simulink model "SpeedgoatCANOpen07"  (R2018b)
settings: Solver=FixedStepDiscrete  StartTime=0.0  StopTime=inf  FixedStep=0.0001  RelTol=1e-3  EnableMultiTasking=on
libraries: slrtlib x9, speedgoatlib_IO691 x5
(part 1 of 2)
settings Model: DataDictionary=Trike_dictionary.sldd  SimulationMode=external  Creator=Venqo  LastModifiedBy=Venqo
settings SolverCC: ConcurrentTasks=on  AutoInsertRateTranBlk=on
settings DataIOCC: SaveFormat=StructureWithTime
settings OptimizationCC: BlockReduction=off  OptimizeBlockIOStorage=off  BufferReuse=off  GlobalBufferReuse=off  ExpressionFolding=off  LocalBlockOutputs=off  RollThreshold=10  OptimizeDataStoreBuffers=off  BusAssignmentInplaceUpdate=off
settings HardwareCC: ProdBitPerPointer=32  ProdBitPerSizeT=32  ProdBitPerPtrDiffT=32  ProdLargestAtomicFloat=None  ProdWordSize=32  ProdLongLongMode=on  ProdHWDeviceType=Generic->32-bit x86 compatible
settings SFSimCC: SimAnalyzeCustomCode=on
settings SFSimCC: SimCustomHeaderCode=|
  | #include "CANOpenSlave.h"
  | #include "CANOpenSlaveAPT.h"
settings SFSimCC: SimCustomInitializer=|
  | CANOpenSlave_ResetCommunication();
  | CANOpenSlave_ResetCommunication_APT();
settings SFSimCC: SimUserSources=|
  | CANOpenSlave.c
  | CANOpenSlaveAPT.c
settings RTWCC: SystemTargetFile=slrt.tlc  TemplateMakefile=slrt_default_tmf  Description=Simulink Real-Time  CodeExecutionProfiling=on  RTWCompilerOptimization=on
settings RTWCC: CustomHeaderCode=|
  | #include "CANOpenSlave.h"
  | #include "CANOpenSlaveAPT.h"
settings RTWCC: CustomSource=|
  | CANOpenSlave.c
  | CANOpenSlaveAPT.c
settings RTWCC: CustomInitializer=|
  | CANOpenSlave_ResetCommunication();
  | CANOpenSlave_ResetCommunication_APT();
settings SimulinkRealTimeCC: InferredTypesCompatibility=on  SupportVariableSizeSignals=on  PreserveStateflowLocalDataDimensions=off  RL32LogTETModifier=off  xPCConcurrentTasks=on

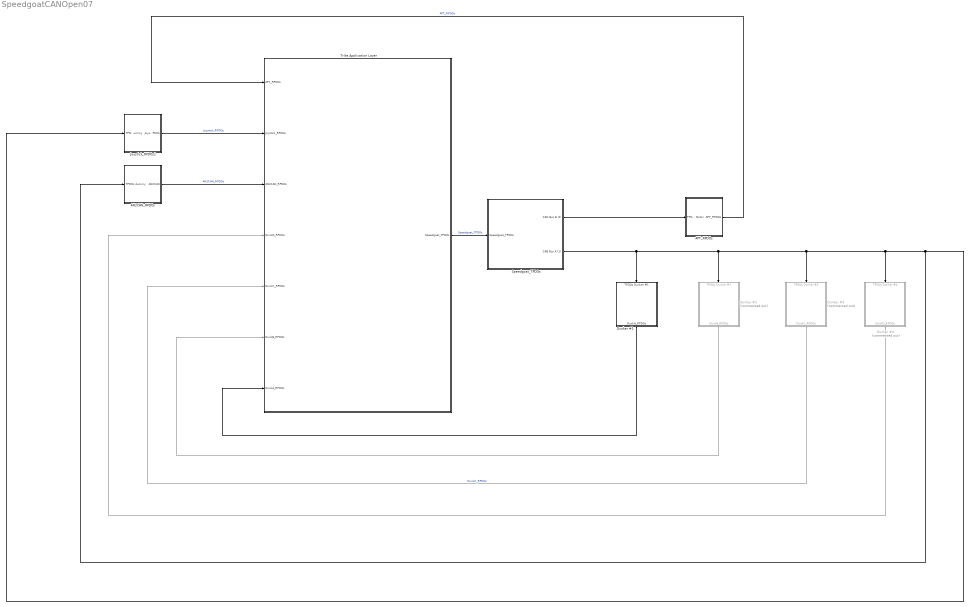
== system SpeedgoatCANOpen07 ==
  AN2CAN_RPDOs : Subsystem
      mask Display: image('C:\Users\Venqo\Desktop\SpeedGoat\Applications\Trike_01_2CANbuses\Img\mcan_box_4xi.png');
  APT_RPDOs : Subsystem
      mask Display: image('C:\Users\Venqo\Desktop\SpeedGoat\Applications\Trike_05\Img\aptqsmotor.png');
  Dunker #1 : Subsystem
      mask Display: image('C:\Users\Venqo\Desktop\SpeedGoat\Applications\Trike_01_2CANbuses\Img\dunk.png');
  Dunker #2 : Subsystem  Commented=on
      mask Display: image('C:\Users\Venqo\Desktop\SpeedGoat\Applications\Trike_01_2CANbuses\Img\dunk.png');
  Dunker #3 : Subsystem  Commented=on
      mask Display: image('C:\Users\Venqo\Desktop\SpeedGoat\Applications\Trike_01_2CANbuses\Img\dunk.png');
  Dunker #4 : Subsystem  Commented=on
      mask Display: image('C:\Users\Venqo\Desktop\SpeedGoat\Applications\Trike_01_2CANbuses\Img\dunk.png');
  Joystick_RPDOs1 : Subsystem
      mask Display: image('C:\Users\Venqo\Desktop\SpeedGoat\Applications\Trike_05\Img\joystick.png');
  Speedgoat_TPDOs : Subsystem
      mask Display: image('C:\Users\Venqo\Desktop\SpeedGoat\Applications\Trike_05\Img\speedgoat.png');
  Trike Application Layer : Subsystem
      mask Display: image('C:\Users\Venqo\Desktop\SpeedGoat\Applications\Trike_05\Img\trike.png');
  wires:
  Joystick_RPDOs1/1(Joystick_RPDOs) -> Trike Application Layer/2(Joystick_RPDOs)  "Joystick_RPDOs"
  Trike Application Layer/1(Speedgoat_TPDOs) -> Speedgoat_TPDOs/1(Speedgoat_TPDOs)  "Speedgoat_TPDOs"
  AN2CAN_RPDOs/1(AN2CAN) -> Trike Application Layer/3(AN2CAN_RPDOs)  "AN2CAN_RPDOs"
  Dunker #3/1(DunkC_RPDOs) -> Trike Application Layer/5(DunkC_RPDOs)  "DunkC_RPDOs"
  Dunker #1/1(DunkA_RPDOs) -> Trike Application Layer/7(DunkA_RPDOs)
  Dunker #2/1(DunkB_RPDOs) -> Trike Application Layer/6(DunkB_RPDOs)
  Dunker #4/1(DunkD_RPDOs) -> Trike Application Layer/4(DunkD_RPDOs)
  Speedgoat_TPDOs/1("CAN Bus B (2) ") -> APT_RPDOs/1("TPDOs APT - QS Motor ")
  APT_RPDOs/1(APT_RPDOs) -> Trike Application Layer/1(APT_RPDOs)  "APT_RPDOs"
  Speedgoat_TPDOs/2(CAB Bus A (1)) -> Dunker #1/1(TPDOs Dunker #1), Dunker #2/1(TPDOs Dunker #1), Dunker #3/1(TPDOs Dunker #3), Dunker #4/1(TPDOs Dunker #4), AN2CAN_RPDOs/1(TPDOs dummy), Joystick_RPDOs1/1(TPDOs dummy)

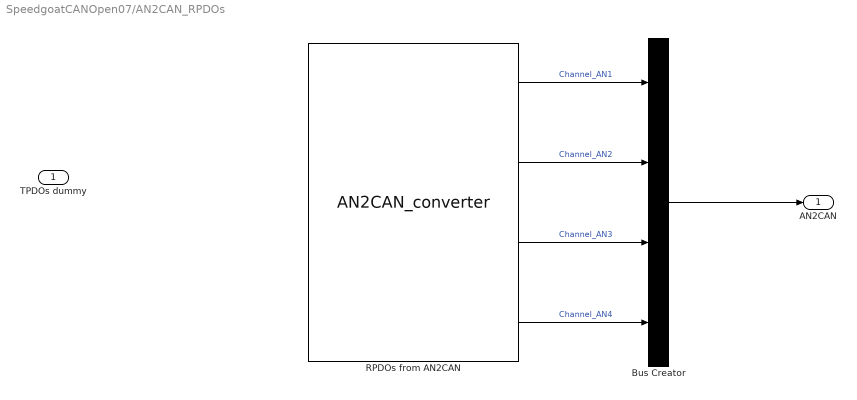
== system SpeedgoatCANOpen07/AN2CAN_RPDOs ==
  TPDOs dummy : Inport
  Bus Creator : BusCreator  Inputs=4  OutDataTypeStr=Bus: AN2CAN_conv
  "RPDOs from AN2CAN " : S-Function  InitFcn=try, set_param(gcb,'FunctionName','AN2CAN_converter'), end  FunctionName=AN2CAN_converter  SFunctionModules=AN2CAN_converter_wrapper  SFunctionDeploymentMode=off  EnableBusSupport=off  mask(S-Function Builder){}
      mask help: Simulink:masks:SFunctionBuilder_MD
      mask init:
      | val = [[.9  0.75 0.75 1 1 .9 .9 1]',[1 1 0.75 0.75 .9 .9 1 .9]'];try , sys = get_param(gcb,'SfunBuilderFcnName');if isempty(sys), sys = get_param(gcb,'FunctionName'); end,catch, sys = get_param(gcb,'FunctionName'); end
      settings: CopyFcn=set_param(gcbh,'LinkStatus','none')  PreSaveFcn=try, set_param(gcb,'FunctionName','AN2CAN_converter'), end  OpenFcn=sfunctionwizard(gcbh)
      mask Display: plot(val(:,1),val(:,2)),disp(sys), port_label('output',1,'Channel_AN1'), port_label('output',2,'Channel_AN2'), port_label('output',3,'Channel_AN3'), port_label('output',4,'Channel_AN4')
  AN2CAN : Outport  OutDataTypeStr=Bus: AN2CAN_conv
  wires:
  Bus Creator/1 -> AN2CAN/1
  "RPDOs from AN2CAN "/3 -> Bus Creator/3  "Channel_AN3"
  "RPDOs from AN2CAN "/4 -> Bus Creator/4  "Channel_AN4"
  "RPDOs from AN2CAN "/2 -> Bus Creator/2  "Channel_AN2"
  "RPDOs from AN2CAN "/1 -> Bus Creator/1  "Channel_AN1"

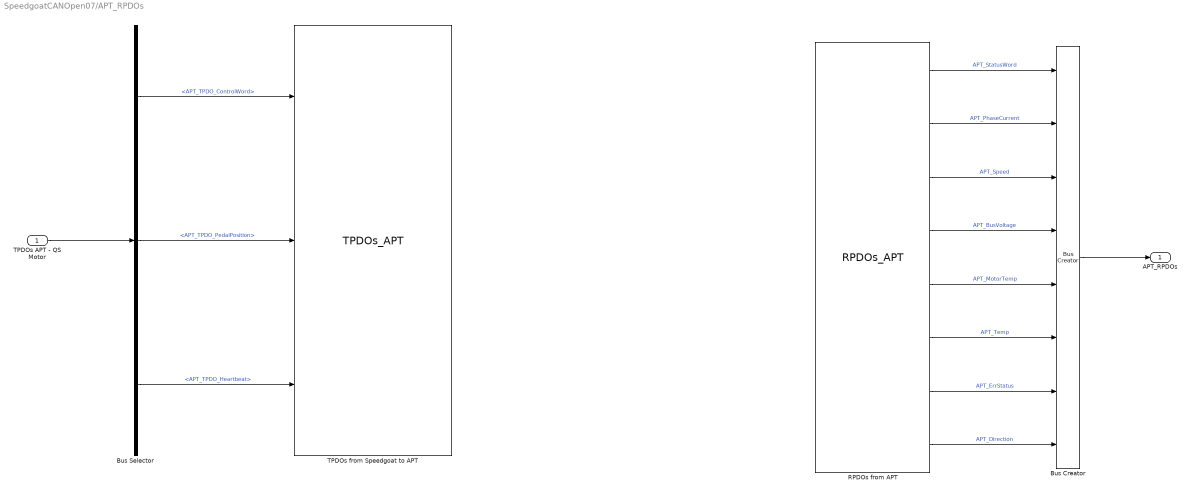
== system SpeedgoatCANOpen07/APT_RPDOs ==
  "TPDOs APT - QS Motor " : Inport
  Bus Creator : BusCreator  Inputs=8  OutDataTypeStr=Bus: APT_RPDOs
  Bus Selector : BusSelector  OutputSignals=APT_TPDO_ControlWord,APT_TPDO_PedalPosition,APT_TPDO_Heartbeat
  RPDOs from APT : S-Function  InitFcn=try, set_param(gcb,'FunctionName','RPDOs_APT'), end  FunctionName=RPDOs_APT  SFunctionModules=RPDOs_APT_wrapper  SFunctionDeploymentMode=off  EnableBusSupport=off  mask(S-Function Builder){}
      mask help: Simulink:masks:SFunctionBuilder_MD
      mask init: same as SpeedgoatCANOpen07/AN2CAN_RPDOs/RPDOs from AN2CAN 
      settings: CopyFcn=set_param(gcbh,'LinkStatus','none')  PreSaveFcn=try, set_param(gcb,'FunctionName','RPDOs_APT'), end  OpenFcn=sfunctionwizard(gcbh)
      mask Display: plot(val(:,1),val(:,2)),disp(sys), port_label('output',1,'StatusWord'), port_label('output',2,'PhaseCurrent'), port_label('output',3,'Speed'), port_label('output',4,'BusVoltage'), port_label('output',5,'MotorTemp'), port_label('output',6,'APTTemp'), port_label('output',7,'ErrStatus'), port_label('output',8,'Direction')
  TPDOs from Speedgoat to APT : S-Function  InitFcn=try, set_param(gcb,'FunctionName','TPDOs_APT'), end  FunctionName=TPDOs_APT  SFunctionModules=TPDOs_APT_wrapper  SFunctionDeploymentMode=off  EnableBusSupport=off  mask(S-Function Builder){}
      mask help: Simulink:masks:SFunctionBuilder_MD
      mask init: same as SpeedgoatCANOpen07/AN2CAN_RPDOs/RPDOs from AN2CAN 
      settings: CopyFcn=set_param(gcbh,'LinkStatus','none')  PreSaveFcn=try, set_param(gcb,'FunctionName','TPDOs_APT'), end  OpenFcn=sfunctionwizard(gcbh)
      mask Display: plot(val(:,1),val(:,2)),disp(sys), port_label('input',1,'APT_ControlWord'), port_label('input',2,'APT_PedalPosition'), port_label('input',3,'APT_HeartBeat')
  APT_RPDOs : Outport  OutDataTypeStr=Bus: APT_RPDOs
  wires:
  Bus Creator/1 -> APT_RPDOs/1
  RPDOs from APT/8 -> Bus Creator/8  "APT_Direction"
  RPDOs from APT/2 -> Bus Creator/2  "APT_PhaseCurrent"
  RPDOs from APT/6 -> Bus Creator/6  "APT_Temp"
  RPDOs from APT/3 -> Bus Creator/3  "APT_Speed"
  RPDOs from APT/1 -> Bus Creator/1  "APT_StatusWord"
  RPDOs from APT/5 -> Bus Creator/5  "APT_MotorTemp"
  RPDOs from APT/7 -> Bus Creator/7  "APT_ErrStatus"
  RPDOs from APT/4 -> Bus Creator/4  "APT_BusVoltage"
  "TPDOs APT - QS Motor "/1 -> Bus Selector/1
  Bus Selector/1 -> TPDOs from Speedgoat to APT/1  "<APT_TPDO_ControlWord>"
  Bus Selector/2 -> TPDOs from Speedgoat to APT/2  "<APT_TPDO_PedalPosition>"
  Bus Selector/3 -> TPDOs from Speedgoat to APT/3  "<APT_TPDO_Heartbeat>"

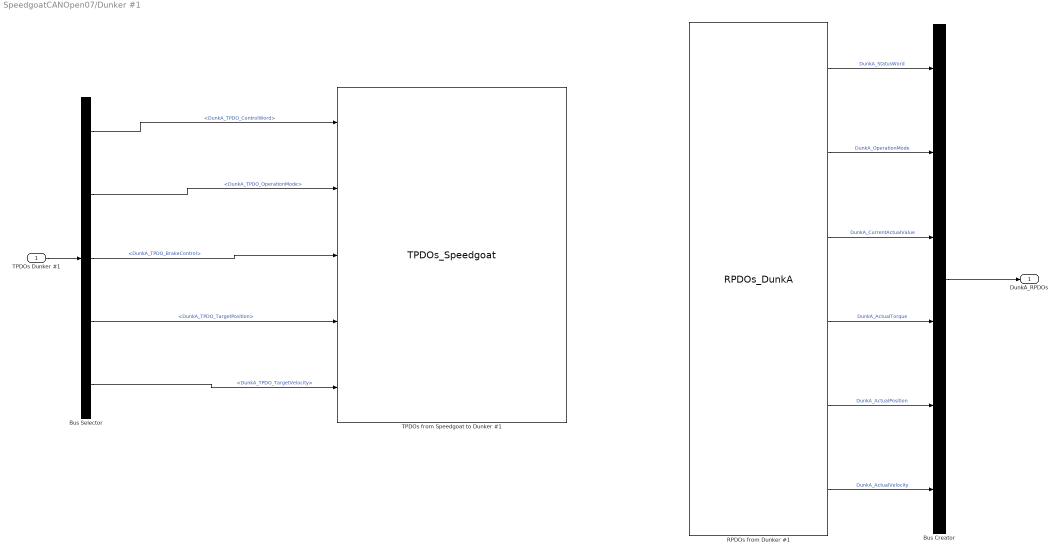
== system SpeedgoatCANOpen07/Dunker #1 ==
  TPDOs Dunker #1 : Inport
  Bus Creator : BusCreator  Inputs=6
  Bus Selector : BusSelector  OutputSignals=DunkA_TPDO_ControlWord,DunkA_TPDO_OperationMode,DunkA_TPDO_BrakeControl,DunkA_TPDO_TargetPosition,DunkA_TPDO_TargetVelocity
  RPDOs from Dunker #1 : S-Function  InitFcn=try, set_param(gcb,'FunctionName','RPDOs_DunkA'), end  FunctionName=RPDOs_DunkA  SFunctionModules=RPDOs_DunkA_wrapper  SFunctionDeploymentMode=off  EnableBusSupport=off  mask(S-Function Builder){}
      mask help: Simulink:masks:SFunctionBuilder_MD
      mask init: same as SpeedgoatCANOpen07/AN2CAN_RPDOs/RPDOs from AN2CAN 
      settings: CopyFcn=set_param(gcbh,'LinkStatus','none')  PreSaveFcn=try, set_param(gcb,'FunctionName','RPDOs_DunkA'), end  OpenFcn=sfunctionwizard(gcbh)
      mask Display: plot(val(:,1),val(:,2)),disp(sys), port_label('output',1,'StatusWord'), port_label('output',2,'OperationMode'), port_label('output',3,'CurrentActualValue'), port_label('output',4,'ActualTorque'), port_label('output',5,'ActualPosition'), port_label('output',6,'ActualVelocity')
  TPDOs from Speedgoat to Dunker #1 : S-Function  InitFcn=try, set_param(gcb,'FunctionName','TPDOs_Speedgoat'), end  FunctionName=TPDOs_Speedgoat  SFunctionModules=TPDOs_Speedgoat_wrapper  SFunctionDeploymentMode=off  EnableBusSupport=off  mask(S-Function Builder){}
      mask help: Simulink:masks:SFunctionBuilder_MD
      mask init: same as SpeedgoatCANOpen07/AN2CAN_RPDOs/RPDOs from AN2CAN 
      settings: CopyFcn=set_param(gcbh,'LinkStatus','none')  PreSaveFcn=try, set_param(gcb,'FunctionName','TPDOs_Speedgoat'), end  OpenFcn=sfunctionwizard(gcbh)
      mask Display: plot(val(:,1),val(:,2)),disp(sys), port_label('input',1,'DunkA_ControlWord'), port_label('input',2,'DunkA_OperationMode'), port_label('input',3,'DunkA_BrakeControl'), port_label('input',4,'DunkA_TargetPosition'), port_label('input',5,'DunkA_TargetVelocity')
  DunkA_RPDOs : Outport
  wires:
  Bus Selector/2 -> TPDOs from Speedgoat to Dunker #1/2  "<DunkA_TPDO_OperationMode>"
  Bus Selector/5 -> TPDOs from Speedgoat to Dunker #1/5  "<DunkA_TPDO_TargetVelocity>"
  TPDOs Dunker #1/1 -> Bus Selector/1
  Bus Selector/4 -> TPDOs from Speedgoat to Dunker #1/4  "<DunkA_TPDO_TargetPosition>"
  Bus Selector/1 -> TPDOs from Speedgoat to Dunker #1/1  "<DunkA_TPDO_ControlWord>"
  Bus Selector/3 -> TPDOs from Speedgoat to Dunker #1/3  "<DunkA_TPDO_BrakeControl>"
  RPDOs from Dunker #1/6 -> Bus Creator/6  "DunkA_ActualVelocity"
  Bus Creator/1 -> DunkA_RPDOs/1
  RPDOs from Dunker #1/1 -> Bus Creator/1  "DunkA_StatusWord"
  RPDOs from Dunker #1/4 -> Bus Creator/4  "DunkA_ActualTorque"
  RPDOs from Dunker #1/2 -> Bus Creator/2  "DunkA_OperationMode"
  RPDOs from Dunker #1/3 -> Bus Creator/3  "DunkA_CurrentActualValue"
  RPDOs from Dunker #1/5 -> Bus Creator/5  "DunkA_ActualPosition"

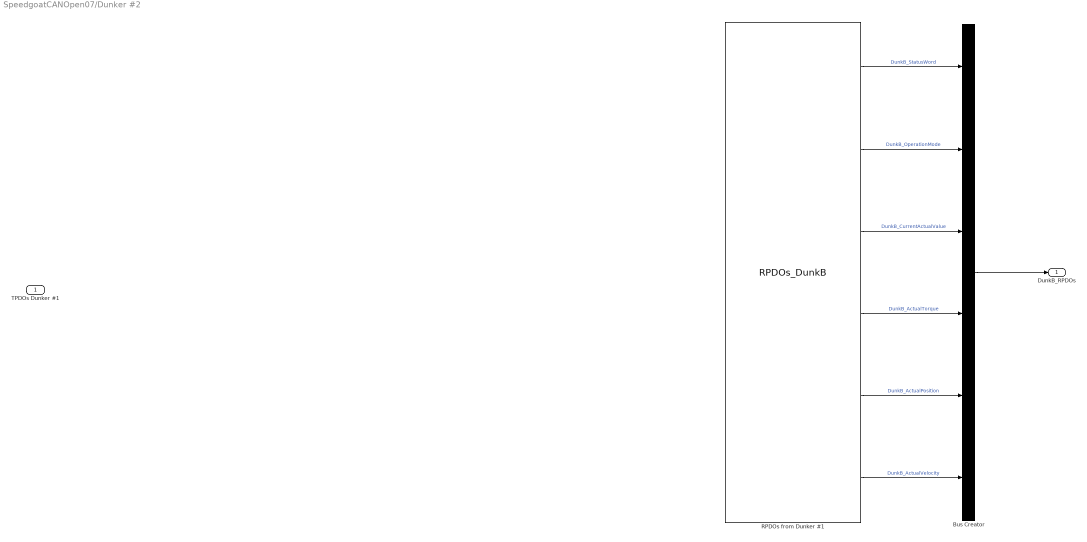
== system SpeedgoatCANOpen07/Dunker #2 ==
  TPDOs Dunker #1 : Inport
  Bus Creator : BusCreator  Inputs=6
  RPDOs from Dunker #1 : S-Function  InitFcn=try, set_param(gcb,'FunctionName','RPDOs_DunkB'), end  FunctionName=RPDOs_DunkB  SFunctionModules=RPDOs_DunkB_wrapper  SFunctionDeploymentMode=off  EnableBusSupport=off  mask(S-Function Builder){}
      mask help: Simulink:masks:SFunctionBuilder_MD
      mask init: same as SpeedgoatCANOpen07/AN2CAN_RPDOs/RPDOs from AN2CAN 
      settings: CopyFcn=set_param(gcbh,'LinkStatus','none')  PreSaveFcn=try, set_param(gcb,'FunctionName','RPDOs_DunkB'), end  OpenFcn=sfunctionwizard(gcbh)
      mask Display: plot(val(:,1),val(:,2)),disp(sys), port_label('output',1,'StatusWord'), port_label('output',2,'OperationMode'), port_label('output',3,'CurrentActualValue'), port_label('output',4,'ActualTorque'), port_label('output',5,'ActualPosition'), port_label('output',6,'ActualVelocity')
  DunkB_RPDOs : Outport
  wires:
  RPDOs from Dunker #1/1 -> Bus Creator/1  "DunkB_StatusWord"
  RPDOs from Dunker #1/3 -> Bus Creator/3  "DunkB_CurrentActualValue"
  RPDOs from Dunker #1/6 -> Bus Creator/6  "DunkB_ActualVelocity"
  RPDOs from Dunker #1/4 -> Bus Creator/4  "DunkB_ActualTorque"
  RPDOs from Dunker #1/5 -> Bus Creator/5  "DunkB_ActualPosition"
  Bus Creator/1 -> DunkB_RPDOs/1
  RPDOs from Dunker #1/2 -> Bus Creator/2  "DunkB_OperationMode"

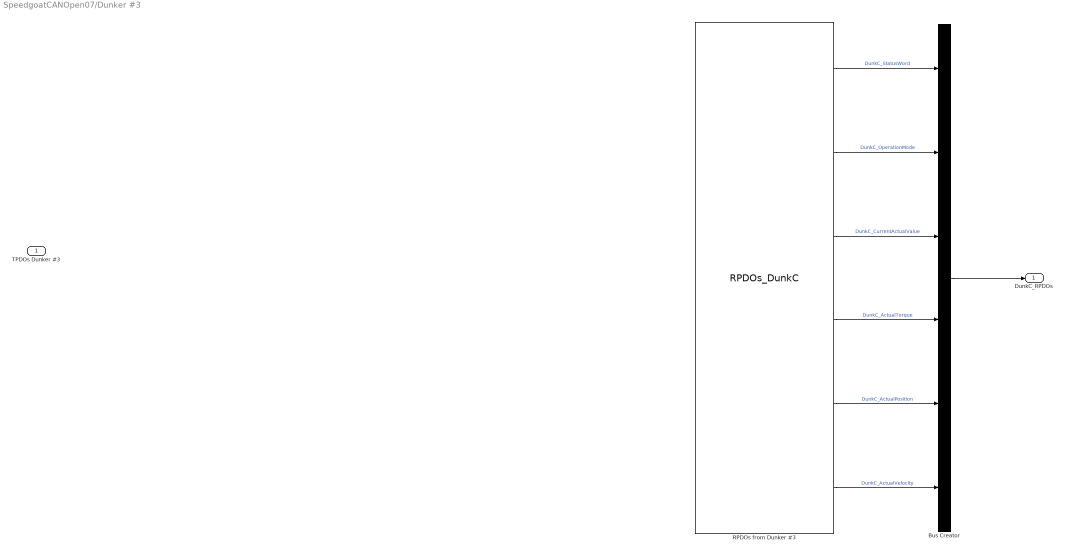
== system SpeedgoatCANOpen07/Dunker #3 ==
  TPDOs Dunker #3 : Inport
  Bus Creator : BusCreator  Inputs=6
  RPDOs from Dunker #3 : S-Function  InitFcn=try, set_param(gcb,'FunctionName','RPDOs_DunkC'), end  FunctionName=RPDOs_DunkC  SFunctionModules=RPDOs_DunkC_wrapper  SFunctionDeploymentMode=off  EnableBusSupport=off  mask(S-Function Builder){}
      mask help: Simulink:masks:SFunctionBuilder_MD
      mask init: same as SpeedgoatCANOpen07/AN2CAN_RPDOs/RPDOs from AN2CAN 
      settings: CopyFcn=set_param(gcbh,'LinkStatus','none')  PreSaveFcn=try, set_param(gcb,'FunctionName','RPDOs_DunkC'), end  OpenFcn=sfunctionwizard(gcbh)
      mask Display: plot(val(:,1),val(:,2)),disp(sys), port_label('output',1,'StatusWord'), port_label('output',2,'OperationMode'), port_label('output',3,'CurrentActualValue'), port_label('output',4,'ActualTorque'), port_label('output',5,'ActualPosition'), port_label('output',6,'ActualVelocity')
  DunkC_RPDOs : Outport
  wires:
  Bus Creator/1 -> DunkC_RPDOs/1
  RPDOs from Dunker #3/3 -> Bus Creator/3  "DunkC_CurrentActualValue"
  RPDOs from Dunker #3/5 -> Bus Creator/5  "DunkC_ActualPosition"
  RPDOs from Dunker #3/4 -> Bus Creator/4  "DunkC_ActualTorque"
  RPDOs from Dunker #3/1 -> Bus Creator/1  "DunkC_StatusWord"
  RPDOs from Dunker #3/2 -> Bus Creator/2  "DunkC_OperationMode"
  RPDOs from Dunker #3/6 -> Bus Creator/6  "DunkC_ActualVelocity"

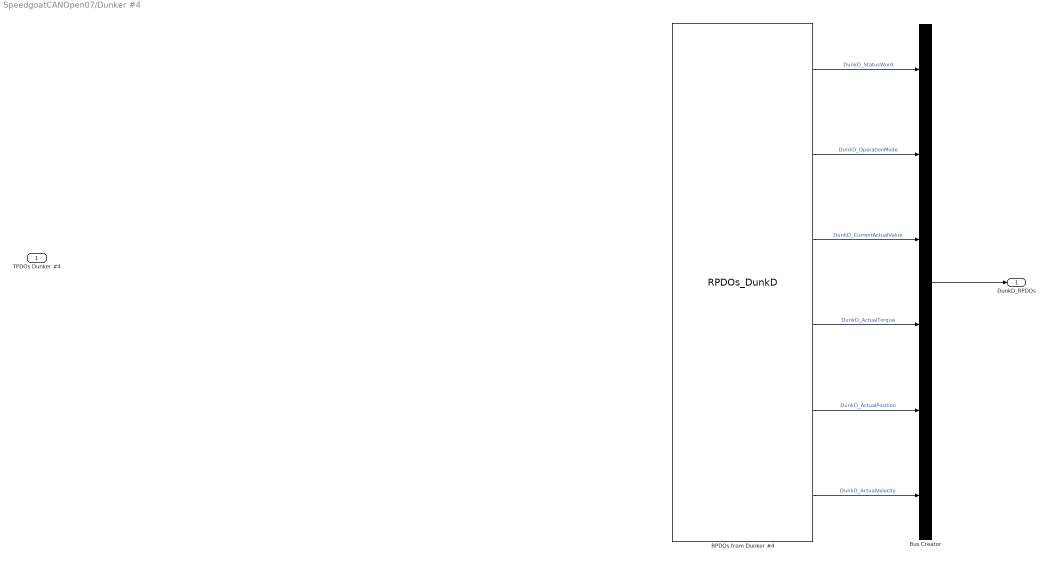
== system SpeedgoatCANOpen07/Dunker #4 ==
  TPDOs Dunker #4 : Inport
  Bus Creator : BusCreator  Inputs=6
  RPDOs from Dunker #4 : S-Function  InitFcn=try, set_param(gcb,'FunctionName','RPDOs_DunkD'), end  FunctionName=RPDOs_DunkD  SFunctionModules=RPDOs_DunkD_wrapper  SFunctionDeploymentMode=off  EnableBusSupport=off  mask(S-Function Builder){}
      mask help: Simulink:masks:SFunctionBuilder_MD
      mask init: same as SpeedgoatCANOpen07/AN2CAN_RPDOs/RPDOs from AN2CAN 
      settings: CopyFcn=set_param(gcbh,'LinkStatus','none')  PreSaveFcn=try, set_param(gcb,'FunctionName','RPDOs_DunkD'), end  OpenFcn=sfunctionwizard(gcbh)
      mask Display: plot(val(:,1),val(:,2)),disp(sys), port_label('output',1,'StatusWord'), port_label('output',2,'OperationMode'), port_label('output',3,'CurrentActualValue'), port_label('output',4,'ActualTorque'), port_label('output',5,'ActualPosition'), port_label('output',6,'ActualVelocity')
  DunkD_RPDOs : Outport
  wires:
  Bus Creator/1 -> DunkD_RPDOs/1
  RPDOs from Dunker #4/1 -> Bus Creator/1  "DunkD_StatusWord"
  RPDOs from Dunker #4/5 -> Bus Creator/5  "DunkD_ActualPosition"
  RPDOs from Dunker #4/4 -> Bus Creator/4  "DunkD_ActualTorque"
  RPDOs from Dunker #4/3 -> Bus Creator/3  "DunkD_CurrentActualValue"
  RPDOs from Dunker #4/6 -> Bus Creator/6  "DunkD_ActualVelocity"
  RPDOs from Dunker #4/2 -> Bus Creator/2  "DunkD_OperationMode"

== system SpeedgoatCANOpen07/Joystick_RPDOs1 ==
  TPDOs dummy : Inport
  Bus Creator : BusCreator  Inputs=3  OutDataTypeStr=Bus: Joystick_RPDOs
  RPDOs from Joystick : S-Function  InitFcn=try, set_param(gcb,'FunctionName','RPDOs_Joystick'), end  FunctionName=RPDOs_Joystick  SFunctionModules=RPDOs_Joystick_wrapper  SFunctionDeploymentMode=off  EnableBusSupport=off  mask(S-Function Builder){}
      mask help: Simulink:masks:SFunctionBuilder_MD
      mask init: same as SpeedgoatCANOpen07/AN2CAN_RPDOs/RPDOs from AN2CAN 
      settings: CopyFcn=set_param(gcbh,'LinkStatus','none')  PreSaveFcn=try, set_param(gcb,'FunctionName','RPDOs_Joystick'), end  OpenFcn=sfunctionwizard(gcbh)
      mask Display: plot(val(:,1),val(:,2)),disp(sys), port_label('output',1,'ButtonsStatus'), port_label('output',2,'LongCmd'), port_label('output',3,'LatCmd')
  Joystick_RPDOs : Outport  OutDataTypeStr=Bus: Joystick_RPDOs
  wires:
  RPDOs from Joystick/3 -> Bus Creator/3  "Joystick_LatCmd"
  RPDOs from Joystick/2 -> Bus Creator/2  "Joystick_LongCmd"
  RPDOs from Joystick/1 -> Bus Creator/1  "Joystick_ButtonsStatus"
  Bus Creator/1 -> Joystick_RPDOs/1

== system SpeedgoatCANOpen07/Speedgoat_TPDOs ==
  Speedgoat_TPDOs : Inport  OutDataTypeStr=Bus: Speedgoat_TPDOs
  CAN Bus Communication : Subsystem
  "CAN Bus B (2) " : Outport
  CAB Bus A (1) : Outport  Port=2
  wires:
  Speedgoat_TPDOs/1 -> CAB Bus A (1)/1, "CAN Bus B (2) "/1

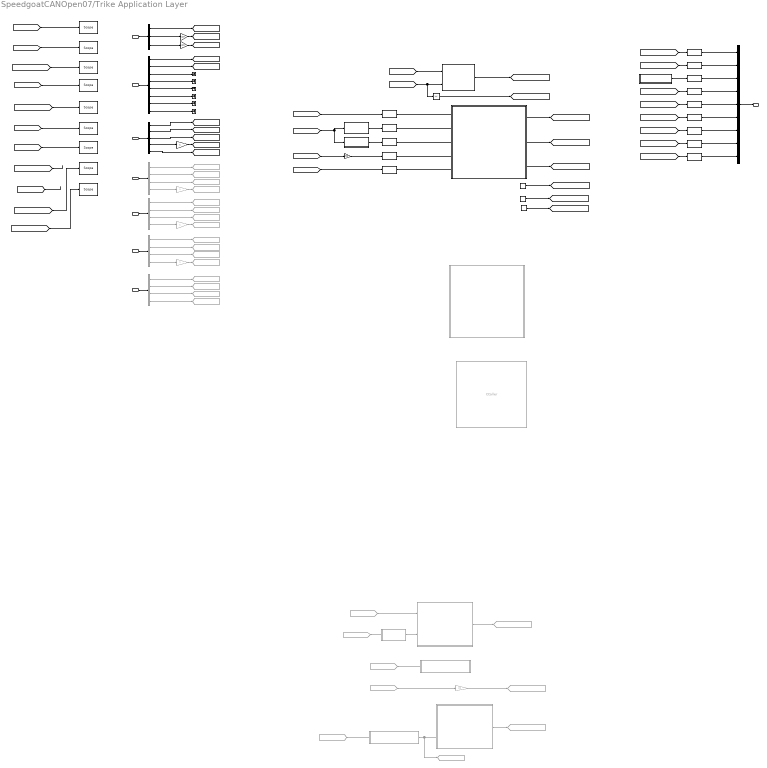
== system SpeedgoatCANOpen07/Trike Application Layer ==
  note: Speedgoat TPDOs / Control
  note: Speedgoat_Scopes
  note: RPDOs from Trike / Feedbacks
  APT_RPDOs : Inport  OutDataTypeStr=Bus: APT_RPDOs
  Joystick_RPDOs : Inport  Port=2  OutDataTypeStr=Bus: Joystick_RPDOs
  AN2CAN_RPDOs : Inport  Port=3  OutDataTypeStr=Bus: AN2CAN_conv
  DunkD_RPDOs : Inport  Port=4
  DunkC_RPDOs : Inport  Port=5
  DunkB_RPDOs : Inport  Port=6
  DunkA_RPDOs : Inport  Port=7
  APT BusVoltage : slrtlib/Displays and Logging/Scope   scopeno=3  scopetype=Target  autostart=on  viewmode=Graphical sliding  formatstr='%15.6f'  grid=on  ylimits=[0,130]  nosamples=50000  noprepostsamples=0  interleave=1  triggermode=FreeRun  triggersignal=1  trigsignalfromport=off  triggerlevel=0.0  triggerslope=Rising  triggerscope=1  triggersample=0  filename=data.dat  mode=Lazy  writesize=512  autorestart=off  dynamicfilemode=off  maxwritefilesize=512*1024^2
  Abs : Abs
  Bus Creator : BusCreator  Inputs=9  OutDataTypeStr=Bus: Speedgoat_TPDOs
  Bus Selector : BusSelector  OutputSignals=Joystick_ButtonsStatus,Joystick_LongCmd,Joystick_LatCmd
  Bus Selector1 : BusSelector  OutputSignals=APT_StatusWord,APT_PhaseCurrent,APT_Speed,APT_BusVoltage,APT_MotorTemp,APT_Temp,APT_ErrStatus,APT_Direction
  Bus Selector2 : BusSelector  OutputSignals=DunkA_StatusWord,DunkA_OperationMode,DunkA_ActualVelocity,DunkA_CurrentActualValue,DunkA_ActualPosition
  Bus Selector3 : BusSelector  Commented=on  OutputSignals=DunkB_StatusWord,DunkB_OperationMode,DunkB_ActualVelocity,DunkB_CurrentActualValue
  Bus Selector4 : BusSelector  Commented=on  OutputSignals=Channel_AN1,Channel_AN2,Channel_AN3,Channel_AN4
  Bus Selector5 : BusSelector  Commented=on  OutputSignals=DunkC_StatusWord,DunkC_OperationMode,DunkC_ActualVelocity,DunkC_CurrentActualValue
  Bus Selector6 : BusSelector  Commented=on  OutputSignals=DunkD_StatusWord,DunkD_OperationMode,DunkD_ActualVelocity,DunkD_CurrentActualValue
  C Caller : CCaller  Commented=on  FunctionName=Position_Control  PortSpecificationStruct="%)30     .    B P   8    (     @         %    \"     @    !     0         %  0 \"0    $    V    07)G3F%M90  4&]R=$YA;64 4V-O<&4     26YD97@     5'EP90      4VEZ90         .    .     8    (    !          %    \"     $    (     0         0    \"    '-T<U]W;W)D#@   #@    &    \"     0         !0    @    !    \"     $         $     @   !S='-?=V]R9 X    X    !@    @    $          4    (     0    4    ! ...(+3947 chars)"
  Constant1 : Constant  Value=0
  Constant2 : Constant  Value=2
  Constant3 : Constant  Value=3000
  Data Type Conversion : DataTypeConversion  OutDataTypeStr=uint8
  Data Type Conversion1 : DataTypeConversion  OutDataTypeStr=uint8
  Data Type Conversion10 : DataTypeConversion  OutDataTypeStr=int8
  Data Type Conversion11 : DataTypeConversion  OutDataTypeStr=int32
  Data Type Conversion{3,9,12..13} (4 alike) : DataTypeConversion  OutDataTypeStr=uint16
  Data Type Conversion2 : DataTypeConversion  OutDataTypeStr=uint8
  Data Type Conversion4 : DataTypeConversion  OutDataTypeStr=int32
  Data Type Conversion5 : DataTypeConversion  OutDataTypeStr=int16
  Data Type Conversion6 : DataTypeConversion  OutDataTypeStr=int8
  Data Type Conversion7 : DataTypeConversion  OutDataTypeStr=int16
  Data Type Conversion8 : DataTypeConversion  OutDataTypeStr=int32
  ElectricDrive_state_machine1 : Stateflow chart  Commented=on  TreatAsAtomicUnit=on
  From11 : From  Commented=on  GotoTag=Joystick_ButtonStatus
  From15 : From  Commented=on  GotoTag=Joystick_ButtonStatus
  From21 : From  Commented=on  GotoTag=Joystick_ButtonStatus
  From22 : From  Commented=on  GotoTag=DunkA_StatusWord
  From7 : From  Commented=on  GotoTag=Joystick_LongCmd
  Gain : Gain  Gain=50
  Gain1 : Gain  Gain=1/10
  Gain2 : Gain  Commented=on
  Gain3 : Gain  Gain=1/10
  Gain4 : Gain  Commented=on
  Gain5 : Gain  Commented=on
  Gain6 : Gain
  Gain8 : Gain  Commented=on  Gain=20  OutDataTypeStr=single
  Goto10 : Goto  Commented=on  GotoTag=DunkB_StatusWord
  Goto11 : Goto  Commented=on  GotoTag=DunkB_OperationMode
  Goto12 : Goto  Commented=on  GotoTag=DunkB_ActualVelocity
  Goto13 : Goto  Commented=on  GotoTag=DunkB_CurrentActualValue
  Goto15 : Goto  Commented=on  GotoTag=DunkA_TPDO_TargetVelocity
  Goto17 : Goto  Commented=on  GotoTag=DunkA_TPDO_NMT
  Goto20 : Goto  Commented=on  GotoTag=DunkA_TPDO_ControlWord
  Goto24 : Goto  Commented=on  GotoTag=button7
  Goto25 : Goto  Commented=on  GotoTag=Channel_AN1
  Goto26 : Goto  Commented=on  GotoTag=Channel_AN2
  Goto27 : Goto  Commented=on  GotoTag=Channel_AN3
  Goto28 : Goto  Commented=on  GotoTag=Channel_AN4
  Goto29 : Goto  Commented=on  GotoTag=DunkC_StatusWord
  Goto30 : Goto  Commented=on  GotoTag=DunkC_OperationMode
  Goto31 : Goto  Commented=on  GotoTag=DunkC_ActualVelocity
  Goto32 : Goto  Commented=on  GotoTag=DunkC_CurrentActualValue
  Goto33 : Goto  Commented=on  GotoTag=DunkD_StatusWord
  Goto34 : Goto  Commented=on  GotoTag=DunkD_OperationMode
  Goto35 : Goto  Commented=on  GotoTag=DunkD_ActualVelocity
  Goto36 : Goto  Commented=on  GotoTag=DunkD_CurrentActualValue
  HeartBeatgenerator : MATLAB Function  TreatAsAtomicUnit=on
  MATLAB Function : MATLAB Function  TreatAsAtomicUnit=on
  MATLAB Function1 : MATLAB Function  Commented=on  TreatAsAtomicUnit=on
  MATLAB Function2 : MATLAB Function  Commented=on  TreatAsAtomicUnit=on
  MATLAB Function4 : MATLAB Function  Commented=on  TreatAsAtomicUnit=on
  MATLAB Function6 : MATLAB Function  TreatAsAtomicUnit=on
  MATLAB Function7 : MATLAB Function  TreatAsAtomicUnit=on
  NMT_state_machine : Stateflow chart  Commented=on  TreatAsAtomicUnit=on
  PedalPosition : slrtlib/Displays and Logging/Scope   scopeno=4  scopetype=Target  autostart=on  viewmode=Graphical sliding  formatstr='%15.6f'  grid=on  ylimits=[0,8]  nosamples=50000  noprepostsamples=0  interleave=1  triggermode=FreeRun  triggersignal=1  trigsignalfromport=off  triggerlevel=0.0  triggerslope=Rising  triggerscope=1  triggersample=0  filename=data.dat  mode=Lazy  writesize=512  autorestart=off  dynamicfilemode=off  maxwritefilesize=512*1024^2
  PedalPosition1 : slrtlib/Displays and Logging/Scope   scopeno=5  scopetype=Target  autostart=on  viewmode=Graphical sliding  formatstr='%15.6f'  grid=on  ylimits=[0,8]  nosamples=50000  noprepostsamples=0  interleave=1  triggermode=FreeRun  triggersignal=1  trigsignalfromport=off  triggerlevel=0.0  triggerslope=Rising  triggerscope=1  triggersample=0  filename=data.dat  mode=Lazy  writesize=512  autorestart=off  dynamicfilemode=off  maxwritefilesize=512*1024^2
  PedalPosition2 : slrtlib/Displays and Logging/Scope   scopeno=6  scopetype=Target  autostart=on  viewmode=Graphical sliding  formatstr='%15.6f'  grid=on  ylimits=[-200,200]  nosamples=50000  noprepostsamples=0  interleave=1  triggermode=FreeRun  triggersignal=1  trigsignalfromport=off  triggerlevel=0.0  triggerslope=Rising  triggerscope=1  triggersample=0  filename=data.dat  mode=Lazy  writesize=512  autorestart=off  dynamicfilemode=off  maxwritefilesize=512*1024^2
  PedalPosition3 : slrtlib/Displays and Logging/Scope   scopeno=2  scopetype=Target  autostart=on  viewmode=Graphical sliding  formatstr='%15.6f'  grid=on  ylimits=[0,6000]  nosamples=50000  noprepostsamples=0  interleave=1  triggermode=FreeRun  triggersignal=1  trigsignalfromport=off  triggerlevel=0.0  triggerslope=Rising  triggerscope=1  triggersample=0  filename=data.dat  mode=Lazy  writesize=512  autorestart=off  dynamicfilemode=off  maxwritefilesize=512*1024^2
  PedalPosition4 : slrtlib/Displays and Logging/Scope   scopeno=7  scopetype=Target  autostart=on  viewmode=Graphical sliding  formatstr='%15.6f'  grid=on  ylimits=[-10000,10000]  nosamples=50000  noprepostsamples=0  interleave=1  triggermode=FreeRun  triggersignal=1  trigsignalfromport=off  triggerlevel=0.0  triggerslope=Rising  triggerscope=1  triggersample=0  filename=data.dat  mode=Lazy  writesize=512  autorestart=off  dynamicfilemode=off  maxwritefilesize=512*1024^2
  PedalPosition5 : slrtlib/Displays and Logging/Scope   scopeno=8  scopetype=Target  autostart=on  viewmode=Graphical sliding  formatstr='%15.6f'  grid=on  ylimits=[-5000,5000]  nosamples=50000  noprepostsamples=0  interleave=1  triggermode=FreeRun  triggersignal=1  trigsignalfromport=off  triggerlevel=0.0  triggerslope=Rising  triggerscope=1  triggersample=0  filename=data.dat  mode=Lazy  writesize=512  autorestart=off  dynamicfilemode=off  maxwritefilesize=512*1024^2
  PedalPosition6 : slrtlib/Displays and Logging/Scope   scopeno=1  scopetype=Target  autostart=on  viewmode=Graphical sliding  formatstr='%15.6f'  grid=on  ylimits=[-5,15]  nosamples=50000  noprepostsamples=0  interleave=1  triggermode=FreeRun  triggersignal=1  trigsignalfromport=off  triggerlevel=0.0  triggerslope=Rising  triggerscope=1  triggersample=0  filename=data.dat  mode=Lazy  writesize=512  autorestart=off  dynamicfilemode=off  maxwritefilesize=512*1024^2
  PedalPosition7 : slrtlib/Displays and Logging/Scope   scopeno=9  scopetype=Target  autostart=on  viewmode=Graphical sliding  formatstr='%15.6f'  grid=on  ylimits=[-200,200]  nosamples=50000  noprepostsamples=0  interleave=1  triggermode=FreeRun  triggersignal=1  trigsignalfromport=off  triggerlevel=0.0  triggerslope=Rising  triggerscope=1  triggersample=0  filename=data.dat  mode=Lazy  writesize=512  autorestart=off  dynamicfilemode=off  maxwritefilesize=512*1024^2
  Set_0_pos_homing : Stateflow chart  TreatAsAtomicUnit=on
  Set_0_pos_homing1 : Stateflow chart  Commented=on  TreatAsAtomicUnit=on
  Terminator{1..6} (6 alike) : Terminator
  Speedgoat_TPDOs : Outport  OutDataTypeStr=Bus: Speedgoat_TPDOs
  wires:
  [Joystick_LongCmd] -> MATLAB Function/2(LongCmd), Abs/1
  MATLAB Function/1(Byte0) -> [APT_ControlWord]
  Abs/1 -> [APT_PedalPosition]
  Data Type Conversion1/1 -> Bus Creator/2  "APT_TPDO_PedalPosition"
  HeartBeatgenerator/1(HB) -> Data Type Conversion2/1
  Data Type Conversion2/1 -> Bus Creator/3  "APT_TPDO_Heartbeat"
  Data Type Conversion3/1 -> Bus Creator/4  "DunkA_TPDO_ControlWord"
  Data Type Conversion5/1 -> Bus Creator/9  "DunkA_TPDO_BrakeControl"
  [Joystick_ButtonStatus] -> MATLAB Function/1(ButtonStatus)
  Joystick_RPDOs/1 -> Bus Selector/1
  Bus Selector/3 -> Gain3/1  "<Joystick_LatCmd>"
  Data Type Conversion/1 -> Bus Creator/1  "APT_TPDO_ControlWord"
  [APT_ControlWord] -> Data Type Conversion/1
  [APT_PedalPosition] -> Data Type Conversion1/1
  Gain1/1 -> [Joystick_LongCmd]
  Gain3/1 -> [Joystick_LatCmd]
  APT_RPDOs/1 -> Bus Selector1/1
  Bus Selector1/1 -> [APT_StatusWord]  "<APT_StatusWord>"
  Bus Selector1/2 -> [APT_PhaseCurrent]  "<APT_PhaseCurrent>"
  Bus Selector1/3 -> Terminator1/1  "<APT_Speed>"
  Bus Selector1/4 -> Terminator2/1  "<APT_BusVoltage>"
  Bus Selector1/5 -> Terminator3/1  "<APT_MotorTemp>"
  Bus Selector1/6 -> Terminator4/1  "<APT_Temp>"
  Bus Selector1/7 -> Terminator5/1  "<APT_ErrStatus>"
  Bus Selector1/8 -> Terminator6/1  "<APT_Direction>"
  DunkA_RPDOs/1 -> Bus Selector2/1
  DunkB_RPDOs/1 -> Bus Selector3/1
  Bus Selector2/2 -> [DunkA_OperationMode]  "<DunkA_OperationMode>"
  Bus Selector2/3 -> [DunkA_ActualVelocity]  "<DunkA_ActualVelocity>"
  Bus Selector2/4 -> Gain6/1  "<DunkA_CurrentActualValue>"
  Bus Selector3/1 -> Goto10/1  "<DunkB_StatusWord>"
  Bus Selector3/2 -> Goto11/1  "<DunkB_OperationMode>"
  Bus Selector3/3 -> Goto12/1  "<DunkB_ActualVelocity>"
  Bus Selector3/4 -> Gain4/1  "<DunkB_CurrentActualValue>"
  Gain6/1 -> [DunkA_CurrentActualValue]
  Gain4/1 -> Goto13/1
  Bus Creator/1 -> Speedgoat_TPDOs/1
  Data Type Conversion4/1 -> Bus Creator/7  "DunkA_TPDO_TargetVelocity"
  From7/1 -> Gain8/1
  Gain8/1 -> Goto15/1
  [DunkA_TPDO_TargetVelocity] -> Data Type Conversion4/1
  Constant2/1 -> [DunkA_TPDO_BrakeControl]
  [DunkA_TPDO_BrakeControl] -> Data Type Conversion5/1
  [DunkA_TPDO_ControlWord] -> Data Type Conversion3/1
  From11/1 -> MATLAB Function2/1(ButtonStatus)
  [DunkA_TPDO_OperationMode] -> Data Type Conversion6/1
  Data Type Conversion6/1 -> Bus Creator/5  "DunkA_TPDO_OperationMode"
  [DunkA_TPDO_TargetTorque] -> Data Type Conversion7/1
  Data Type Conversion7/1 -> Bus Creator/6  "DunkA_TPDO_TargetTorque"
  [DunkA_TPDO_TargetPosition] -> Data Type Conversion8/1
  Data Type Conversion8/1 -> Bus Creator/8  "DunkA_TPDO_TargetPosition"
  Bus Selector2/1 -> [DunkA_StatusWord]  "<DunkA_StatusWord>"
  [DunkA_CurrentActualValue] -> PedalPosition6/1  "DunkA_CurrentActualValue"
  [DunkA_TPDO_ControlWord] -> APT BusVoltage/1  "DunkA_TPDO_ControlWord"
  [DunkA_OperationMode] -> PedalPosition/1  "DunkA_OperationMode"
  [DunkA_TPDO_OperationMode] -> PedalPosition1/1  "DunkA_TPDO_OperationMode"
  [Joystick_LatCmd] -> PedalPosition2/1  "Joystick_LatCmd"
  Bus Selector/1 -> [Joystick_ButtonStatus]  "<Joystick_ButtonsStatus>"
  Bus Selector/2 -> Gain1/1  "<Joystick_LongCmd>"
  NMT_state_machine/1(Control) -> Goto17/1
  [DunkA_StatusWord] -> PedalPosition3/1  "DunkA_StatusWord"
  From15/1 -> MATLAB Function1/1(ButtonStatus)
  MATLAB Function1/1(B7) -> Goto24/1, NMT_state_machine/2(PowerOn)
  [DunkA_TPDO_TargetPosition] -> ?  "DunkA_TPDO_TargetPosition"
  MATLAB Function4/1(Byte0) -> ElectricDrive_state_machine1/2(PowerOn)
  From21/1 -> MATLAB Function4/1(ButtonStatus)
  From22/1 -> ElectricDrive_state_machine1/1(StatusWord)
  ElectricDrive_state_machine1/1(ControlWord) -> Goto20/1
  AN2CAN_RPDOs/1 -> Bus Selector4/1
  Bus Selector4/4 -> Goto28/1  "<Channel_AN4>"
  Bus Selector4/3 -> Goto27/1  "<Channel_AN3>"
  Bus Selector4/2 -> Goto26/1  "<Channel_AN2>"
  Bus Selector4/1 -> Goto25/1  "<Channel_AN1>"
  DunkC_RPDOs/1 -> Bus Selector5/1
  Bus Selector5/4 -> Gain2/1  "<DunkC_CurrentActualValue>"
  Bus Selector5/3 -> Goto31/1  "<DunkC_ActualVelocity>"
  Gain2/1 -> Goto32/1
  Bus Selector5/2 -> Goto30/1  "<DunkC_OperationMode>"
  Bus Selector5/1 -> Goto29/1  "<DunkC_StatusWord>"
  DunkD_RPDOs/1 -> Bus Selector6/1
  Bus Selector6/4 -> Gain5/1  "<DunkD_CurrentActualValue>"
  Bus Selector6/3 -> Goto35/1  "<DunkD_ActualVelocity>"
  Gain5/1 -> Goto36/1
  Bus Selector6/2 -> Goto34/1  "<DunkD_OperationMode>"
  Bus Selector6/1 -> Goto33/1  "<DunkD_StatusWord>"
  [DunkA_ActualPosition] -> PedalPosition4/1  "DunkA_ActualPosition"
  Bus Selector2/5 -> [DunkA_ActualPosition]  "<DunkA_ActualPosition>"
  Set_0_pos_homing/1(ControlWord) -> [DunkA_TPDO_ControlWord]  "ctrl_word"
  MATLAB Function6/1(B8) -> Data Type Conversion12/1
  [Joystick_ButtonStatus] -> MATLAB Function7/1(ButtonStatus), MATLAB Function6/1(ButtonStatus)
  MATLAB Function7/1(B7) -> Data Type Conversion13/1
  [DunkA_OperationMode] -> Data Type Conversion10/1
  Set_0_pos_homing/3(TargetPosition) -> [DunkA_TPDO_TargetPosition]  "ctrl_position"
  Gain/1 -> Data Type Conversion11/1
  [Joystick_LongCmd] -> Gain/1
  Set_0_pos_homing/2(OpMode) -> [DunkA_TPDO_OperationMode]  "ctrl_op_mode"
  [DunkA_StatusWord] -> Data Type Conversion9/1
  Data Type Conversion9/1 -> Set_0_pos_homing/1(StatusWord)  "sts_word"
  Data Type Conversion10/1 -> Set_0_pos_homing/5(StatusOpMode)  "sts_op_mode"
  Data Type Conversion11/1 -> Set_0_pos_homing/4(Target)  "target_pos"
  Data Type Conversion12/1 -> Set_0_pos_homing/2(PowerOn)  "poweron"
  Data Type Conversion13/1 -> Set_0_pos_homing/3(B7)  "set_homing"
  Constant3/1 -> [DunkA_TPDO_TargetVelocity]
  [Joystick_LongCmd] -> ?  "Joystick_LongCmd"
  Constant1/1 -> [DunkA_TPDO_TargetTorque]
  [APT_PedalPosition] -> PedalPosition7/1
  [APT_ControlWord] -> PedalPosition5/1

== system SpeedgoatCANOpen07/Speedgoat_TPDOs/CAN Bus Communication ==
  "CAN Setup " : speedgoatlib_IO691/CAN Setup   moduletype=IO691  id=1  pciSlot=-1  chn1=CAN (HS)  chn2=CAN (HS)  chn3=Disabled  chn4=Disabled  initStruct=[]  termStruct=[]  ArbitrationbdrChn1=500 kBaud  ArbitrationManbdrChn1=[2,16,63,16]  FdbdrChn1=5.0 MBaud  FdManbdrChn1=[2,2,5,2]  ArbitrationbdrChn2=500 kBaud  ArbitrationManbdrChn2=[2,16,63,16]  FdbdrChn2=5.0 MBaud  FdManbdrChn2=[2,2,5,2]  ArbitrationbdrChn3=1.0 MBaud  ArbitrationManbdrChn3=[2,8,31,8]  FdbdrChn3=5.0 MBaud  FdManbdrChn3=[2,2,5,2]  ArbitrationbdrChn4=1.0 MBaud  ArbitrationManbdrChn4=[2,8,31,8]  FdbdrChn4=5.0 MBaud  FdManbdrChn4=[2,2,5,2]  moduleInitValues=[691 1 -1 -1]
      settings: SourceProductName=Simulink Real-Time: Speedgoat Library
  CANOpen Slave Protocol Stack - CAN Bus #1 (A) : Subsystem  mask{Ts=0.0001}
      mask prompts: Ts "Sample Time (s)"
      mask Display: disp('CANOpen Slave Stack')
  CANOpen Slave Protocol Stack - CAN Bus #2 (B) : Subsystem  mask{Ts=0.0001}
      mask prompts: Ts "Sample Time (s)"
      mask Display: disp('CANOpen Slave Stack')

== system SpeedgoatCANOpen07/Speedgoat_TPDOs/CAN Bus Communication/CANOpen Slave Protocol Stack - CAN Bus #1 (A) ==
  C Caller : CCaller  FunctionName=CANOpenSlave_ProcessStack  PortSpecificationStruct="%)30     .    ( D   8    (     @         %    \"     8    !     0         %  0 \"0    $    V    07)G3F%M90  4&]R=$YA;64 4V-O<&4     26YD97@     5'EP90      4VEZ90         .    ,     8    (    !          %    \"     $    $     0         0  0 <GA)1 X    P    !@    @    $          4    (     0    0    !         !  ! !R>$E$#@   #@    &    \"     0         !0    @    !    !0    $         $     4   !);G ...(+2763 chars)"
  CAN RX Wrapper : Subsystem
  CAN TX Wrapper : Subsystem
  wires:
  C Caller/2 -> CAN TX Wrapper/Enable, CAN TX Wrapper/2(DLC)
  CAN RX Wrapper/1(ID) -> C Caller/1
  C Caller/1 -> CAN TX Wrapper/1(ID)
  CAN RX Wrapper/2(DLC) -> C Caller/2
  C Caller/3 -> CAN TX Wrapper/3(DATA)
  CAN RX Wrapper/3(DATA) -> C Caller/3

== system SpeedgoatCANOpen07/Speedgoat_TPDOs/CAN Bus Communication/CANOpen Slave Protocol Stack - CAN Bus #2 (B) ==
  C Caller : CCaller  FunctionName=CANOpenSlave_ProcessStack_APT  PortSpecificationStruct="%)30     .    ( D   8    (     @         %    \"     8    !     0         %  0 \"0    $    V    07)G3F%M90  4&]R=$YA;64 4V-O<&4     26YD97@     5'EP90      4VEZ90         .    ,     8    (    !          %    \"     $    $     0         0  0 <GA)1 X    P    !@    @    $          4    (     0    0    !         !  ! !R>$E$#@   #@    &    \"     0         !0    @    !    !0    $         $     4   !);G ...(+2763 chars)"
  CAN RX Wrapper : Subsystem
  CAN TX Wrapper : Subsystem
  wires:
  CAN RX Wrapper/3(DATA) -> C Caller/3
  C Caller/3 -> CAN TX Wrapper/3(DATA)
  CAN RX Wrapper/2(DLC) -> C Caller/2
  C Caller/1 -> CAN TX Wrapper/1(ID)
  CAN RX Wrapper/1(ID) -> C Caller/1
  C Caller/2 -> CAN TX Wrapper/2(DLC), CAN TX Wrapper/Enable

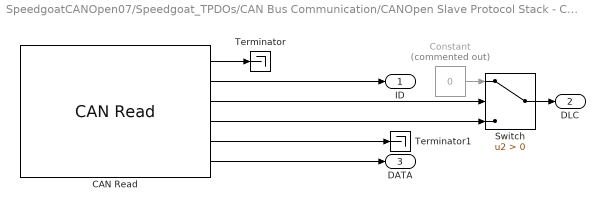
== system SpeedgoatCANOpen07/Speedgoat_TPDOs/CAN Bus Communication/CANOpen Slave Protocol Stack - CAN Bus #1 (A)/CAN RX Wrapper ==
  CAN Read : speedgoatlib_IO691/CAN Read  id=1  ts=Ts  channel=1  messageType=RAW  canType=CAN (HS)  initValues=[691 1 0.0001 0 2 1]
      settings: SourceProductName=Simulink Real-Time: Speedgoat Library
  Constant : Constant  Commented=on  Value=0  OutDataTypeStr=Inherit: Inherit via back propagation
  Switch : Switch  Criteria=u2 > Threshold
  Terminator : Terminator
  Terminator1 : Terminator
  ID : Outport
  DLC : Outport  Port=2
  DATA : Outport  Port=3
  wires:
  CAN Read/4 -> Switch/3
  CAN Read/5 -> Terminator1/1
  Switch/1 -> DLC/1
  CAN Read/2 -> ID/1
  CAN Read/3 -> Switch/2
  CAN Read/6 -> DATA/1
  Constant/1 -> Switch/1
  CAN Read/1 -> Terminator/1

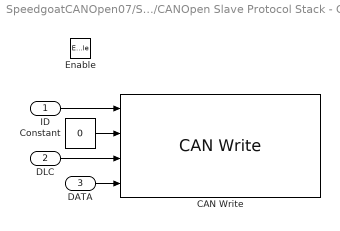
== system SpeedgoatCANOpen07/Speedgoat_TPDOs/CAN Bus Communication/CANOpen Slave Protocol Stack - CAN Bus #1 (A)/CAN TX Wrapper ==
  ID : Inport
  DLC : Inport  Port=2
  DATA : Inport  Port=3
  Enable : EnablePort
  CAN Write : speedgoatlib_IO691/CAN Write  id=1  ts=Ts  channel=1  messageType=RAW  enableStatusPort=off  canType=CAN (HS)  initValues=[691 1 0.0001 0 2 1 0]
      settings: SourceProductName=Simulink Real-Time: Speedgoat Library
  Constant : Constant  Value=0  OutDataTypeStr=Inherit: Inherit via back propagation
  wires:
  ID/1 -> CAN Write/1
  DATA/1 -> CAN Write/4
  DLC/1 -> CAN Write/3
  Constant/1 -> CAN Write/2

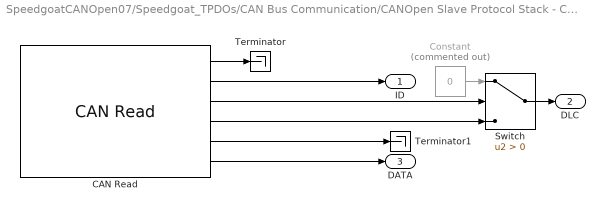
== system SpeedgoatCANOpen07/Speedgoat_TPDOs/CAN Bus Communication/CANOpen Slave Protocol Stack - CAN Bus #2 (B)/CAN RX Wrapper ==
  CAN Read : speedgoatlib_IO691/CAN Read  id=1  ts=Ts  channel=2  messageType=RAW  canType=CAN (HS)  initValues=[691 1 0.0001 1 2 1]
      settings: SourceProductName=Simulink Real-Time: Speedgoat Library
  Constant : Constant  Commented=on  Value=0  OutDataTypeStr=Inherit: Inherit via back propagation
  Switch : Switch  Criteria=u2 > Threshold
  Terminator : Terminator
  Terminator1 : Terminator
  ID : Outport
  DLC : Outport  Port=2
  DATA : Outport  Port=3
  wires:
  CAN Read/1 -> Terminator/1
  Constant/1 -> Switch/1
  CAN Read/6 -> DATA/1
  CAN Read/3 -> Switch/2
  CAN Read/2 -> ID/1
  Switch/1 -> DLC/1
  CAN Read/5 -> Terminator1/1
  CAN Read/4 -> Switch/3

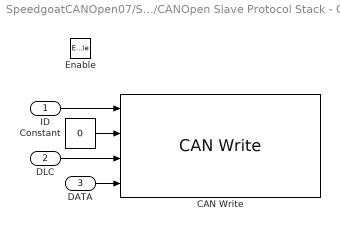
== system SpeedgoatCANOpen07/Speedgoat_TPDOs/CAN Bus Communication/CANOpen Slave Protocol Stack - CAN Bus #2 (B)/CAN TX Wrapper ==
  ID : Inport
  DLC : Inport  Port=2
  DATA : Inport  Port=3
  Enable : EnablePort
  CAN Write : speedgoatlib_IO691/CAN Write  id=1  ts=Ts  channel=2  messageType=RAW  enableStatusPort=off  canType=CAN (HS)  initValues=[691 1 0.0001 1 2 1 0]
      settings: SourceProductName=Simulink Real-Time: Speedgoat Library
  Constant : Constant  Value=0  OutDataTypeStr=Inherit: Inherit via back propagation
  wires:
  Constant/1 -> CAN Write/2
  DLC/1 -> CAN Write/3
  DATA/1 -> CAN Write/4
  ID/1 -> CAN Write/1

== matlab function SpeedgoatCANOpen07/Trike Application Layer/HeartBeatgenerator ==
  data: HB output
function HB = HBGenerator
persistent tact Heartbeat
if (isempty(Heartbeat))
    Heartbeat = 0;
    tact = 0;
end
tact=tact+1;
if (tact>10)
    tact=0;
    Heartbeat=Heartbeat+1;
    if (Heartbeat>127)
        Heartbeat = 0;    
    end
end
HB = Heartbeat;

== matlab function SpeedgoatCANOpen07/Trike Application Layer/MATLAB Function ==
  data: ButtonStatus input; Byte0 output; LongCmd input
function Byte0 = TractionCtrl(ButtonStatus, LongCmd)
Direction =0;
if (ButtonStatus>=127)
    if(LongCmd>0)
        Direction = 4;
    elseif (LongCmd<0)
        Direction = 8;
    end
 end
Byte0 =160+Direction;

== stateflow chart SpeedgoatCANOpen07/Trike Application Layer/NMT_state_machine ==
  state Init
    entry:
    x00s=129;  % 81h
    x00=0;        % h
    x01s=130;  % 82h
    x01=0;        % h
    x1s=127;    % 7Fh
    x1=0;          % h
    x2s=5;        % 05h
    x2=0;          % h
    x3s=4;        % 04h
    x3=0;          % h
    t=3;
  state ResetApplication
    entry:
    Control=x1;
  state ResetCommunication
    entry:
    Control=x2;
  state PreOperational
    entry:
    Control=x3;
  state Operational
    entry:
    Control=x4;
  state Stopped
    entry:
    Control=x5;
  (default) -> Init
  Init -> ResetApplication
  ResetApplication -> ResetCommunication : [PowerOn==1]{after(t,sec)}
  ResetCommunication -> PreOperational : [ PowerOn==1]{after(t,sec)}
  PreOperational -> Operational [order 1] : [PowerOn==1]{after(t,sec)}
  PreOperational -> ResetCommunication [order 3]
  Operational -> PreOperational [order 2]
  PreOperational -> ResetApplication [order 4]
  Stopped -> ResetApplication [order 4]
  Operational -> ResetApplication [order 4]
  Stopped -> ResetCommunication [order 3]
  Operational -> ResetCommunication [order 3]
  Stopped -> PreOperational [order 2]
  PreOperational -> Stopped [order 2]
  Stopped -> Operational [order 1]
  Operational -> Stopped [order 1] : [PowerOn==0]{after(t,sec)}
  data: Status input; PowerOn input; Control output; x1 local; x2 local; x3 local; x00 local; x01 local; x1s local; x2s local; x3s local; x00s local; x01s local; t local

== matlab function SpeedgoatCANOpen07/Trike Application Layer/MATLAB Function2 ==
  data: ButtonStatus input; B8 output
function B8 = Button8Check(ButtonStatus)
aux =1;
if (ButtonStatus==128)
        aux = 2;
else 
    aux =1;
 end
B8 =aux;
